simulink model "add_entry_model"  (R2020b)
settings: Solver=FixedStepDiscrete  StartTime=0.0  StopTime=0.1  FixedStep=0.1  RelTol=1e-3
undefined symbols (not defined in the file or in its folder): kConsecutiveIndexDelta, kContainerLength, test_input
libraries: move_index_lib x2
settings Model: Creator=rsub  LastModifiedBy=rsub

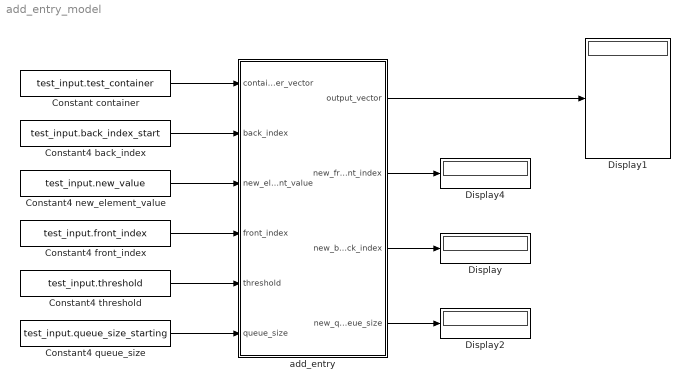
== system add_entry_model ==
  Constant container : Constant  Value=test_input.test_container
  Constant4 back_index : Constant  Value=test_input.back_index_start
  Constant4 front_index : Constant  Value=test_input.front_index
  Constant4 new_element_value : Constant  Value=test_input.new_value
  Constant4 queue_size : Constant  Value=test_input.queue_size_starting
  Constant4 threshold : Constant  Value=test_input.threshold
  Display{,1..2,4} (4 alike) : Display
  add_entry : Subsystem
  wires:
  Constant container/1 -> add_entry/1(container_vector)
  Constant4 back_index/1 -> add_entry/2(back_index)
  Constant4 new_element_value/1 -> add_entry/3(new_element_value)
  add_entry/1(output_vector) -> Display1/1
  add_entry/3(new_back_index) -> Display/1
  Constant4 front_index/1 -> add_entry/4(front_index)
  Constant4 threshold/1 -> add_entry/5(threshold)
  Constant4 queue_size/1 -> add_entry/6(queue_size)
  add_entry/2(new_front_index) -> Display4/1
  add_entry/4(new_queue_size) -> Display2/1

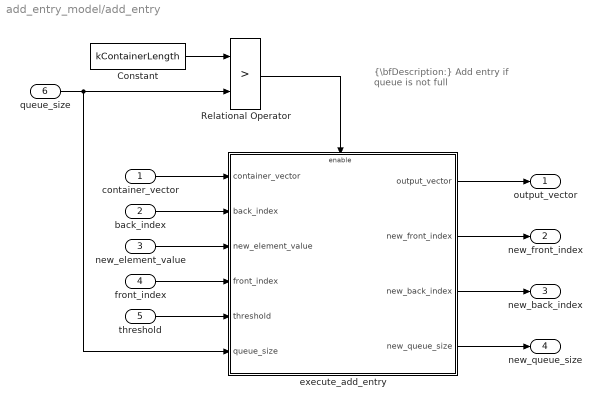
== system add_entry_model/add_entry ==
  note: {\bfDescription:}
      | Add entry if queue is not full
  container_vector : Inport
  back_index : Inport  Port=2
  new_element_value : Inport  Port=3
  front_index : Inport  Port=4
  threshold : Inport  Port=5
  queue_size : Inport  Port=6
  Constant : Constant  Value=kContainerLength
  Relational Operator : RelationalOperator  Operator=>  OutDataTypeStr=boolean  RndMeth=Simplest
  execute_add_entry : Subsystem
  output_vector : Outport
  new_front_index : Outport  Port=2
  new_back_index : Outport  Port=3
  new_queue_size : Outport  Port=4
  wires:
  container_vector/1 -> execute_add_entry/1(container_vector)
  back_index/1 -> execute_add_entry/2(back_index)
  new_element_value/1 -> execute_add_entry/3(new_element_value)
  front_index/1 -> execute_add_entry/4(front_index)
  threshold/1 -> execute_add_entry/5(threshold)
  queue_size/1 -> execute_add_entry/6(queue_size), Relational Operator/2
  execute_add_entry/1(output_vector) -> output_vector/1
  execute_add_entry/2(new_front_index) -> new_front_index/1
  execute_add_entry/3(new_back_index) -> new_back_index/1
  execute_add_entry/4(new_queue_size) -> new_queue_size/1
  Constant/1 -> Relational Operator/1
  Relational Operator/1 -> execute_add_entry/Enable

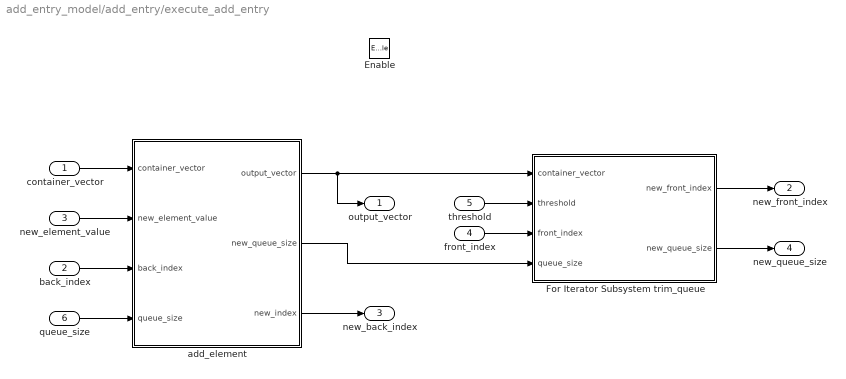
== system add_entry_model/add_entry/execute_add_entry ==
  container_vector : Inport
  back_index : Inport  Port=2
  new_element_value : Inport  Port=3
  front_index : Inport  Port=4
  threshold : Inport  Port=5
  queue_size : Inport  Port=6
  Enable : EnablePort
  For Iterator Subsystem trim_queue : Subsystem  TreatAsAtomicUnit=on
  add_element : Subsystem
  output_vector : Outport  InitialOutput=test_input.test_container
  new_front_index : Outport  Port=2  InitialOutput=test_input.front_index
  new_back_index : Outport  Port=3  InitialOutput=test_input.back_index_start
  new_queue_size : Outport  Port=4  InitialOutput=test_input.queue_size_starting
  wires:
  threshold/1 -> For Iterator Subsystem trim_queue/2(threshold)
  new_element_value/1 -> add_element/2(new_element_value)
  For Iterator Subsystem trim_queue/1(new_front_index) -> new_front_index/1
  container_vector/1 -> add_element/1(container_vector)
  add_element/3(new_index) -> new_back_index/1
  back_index/1 -> add_element/3(back_index)
  front_index/1 -> For Iterator Subsystem trim_queue/3(front_index)
  add_element/2(new_queue_size) -> For Iterator Subsystem trim_queue/4(queue_size)
  For Iterator Subsystem trim_queue/2(new_queue_size) -> new_queue_size/1
  queue_size/1 -> add_element/4(queue_size)
  add_element/1(output_vector) -> output_vector/1, For Iterator Subsystem trim_queue/1(container_vector)

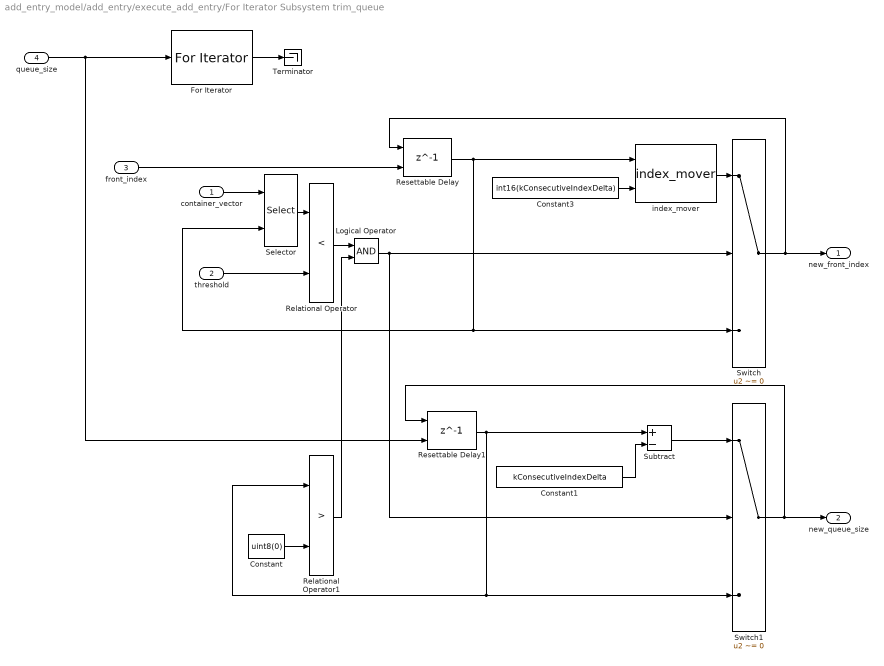
== system add_entry_model/add_entry/execute_add_entry/For Iterator Subsystem trim_queue ==
  container_vector : Inport
  threshold : Inport  Port=2
  front_index : Inport  Port=3
  queue_size : Inport  Port=4
  Constant : Constant  Value=uint8(0)
  Constant1 : Constant  Value=kConsecutiveIndexDelta
  Constant3 : Constant  Value=int16(kConsecutiveIndexDelta)
  For Iterator : ForIterator  IterationSource=external  IterationLimit=kContainerLength  IndexMode=Zero-based  IterationVariableDataType=uint8
  Logical Operator : Logic  AllPortsSameDT=off  OutDataTypeStr=boolean
  Relational Operator : RelationalOperator  Operator=<  OutDataTypeStr=boolean  RndMeth=Simplest
  Relational Operator1 : RelationalOperator  Operator=>  OutDataTypeStr=boolean  RndMeth=Simplest
  Resettable Delay : Delay  DelayLength=1  InitialConditionSource=Input port
      settings: InputPortMap=u0,p4
  Resettable Delay1 : Delay  DelayLength=1  InitialConditionSource=Input port
      settings: InputPortMap=u0,p4
  Selector : Selector  IndexMode=Zero-based  InputPortWidth=kContainerLength  IndexOptions=Index vector (port)  Indices=[1 3]  OutputSizes=1
  Subtract : Sum  Inputs=+-
  Switch : Switch  Criteria=u2 ~= 0
  Switch1 : Switch  Criteria=u2 ~= 0
  Terminator : Terminator
  index_mover : move_index_lib/index_mover  SystemSampleTime=-1  VariantActivationTime=update diagram  Latency=0  AutoFrameSizeCalculation=off
  new_front_index : Outport
  new_queue_size : Outport  Port=2
  wires:
  queue_size/1 -> Resettable Delay1/2, For Iterator/1
  For Iterator/1 -> Terminator/1
  container_vector/1 -> Selector/1
  front_index/1 -> Resettable Delay/2
  Selector/1 -> Relational Operator/1
  threshold/1 -> Relational Operator/2
  Logical Operator/1 -> Switch/2, Switch1/2
  Switch/1 -> Resettable Delay/1, new_front_index/1
  index_mover/1 -> Switch/1
  Constant3/1 -> index_mover/2
  Resettable Delay/1 -> Switch/3, Selector/2, index_mover/1
  Switch1/1 -> new_queue_size/1, Resettable Delay1/1
  Resettable Delay1/1 -> Switch1/3, Relational Operator1/1, Subtract/1
  Subtract/1 -> Switch1/1
  Constant1/1 -> Subtract/2
  Relational Operator/1 -> Logical Operator/1
  Constant/1 -> Relational Operator1/2
  Relational Operator1/1 -> Logical Operator/2

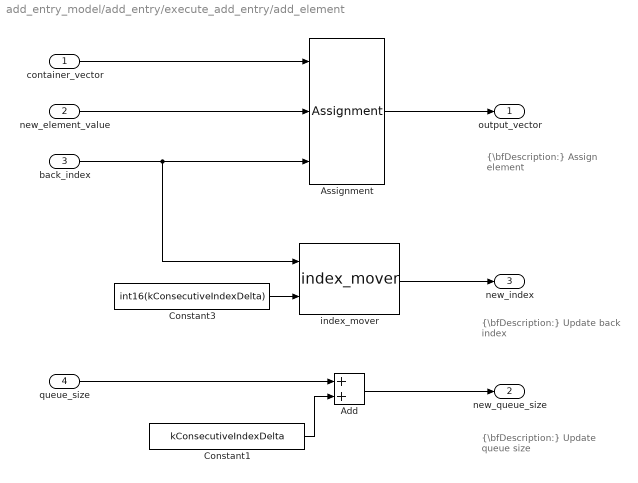
== system add_entry_model/add_entry/execute_add_entry/add_element ==
  note: {\bfDescription:}
      | Assign element
  note: {\bfDescription:}
      | Update back index
  note: {\bfDescription:}
      | Update queue size
  container_vector : Inport
  new_element_value : Inport  Port=2
  back_index : Inport  Port=3
  queue_size : Inport  Port=4
  Add : Sum
  Assignment : Assignment  IndexMode=Zero-based  DiagnosticForDimensions=Warning  IndexOptions=Index vector (port)  Indices=1  OutputSizes=1
  Constant1 : Constant  Value=kConsecutiveIndexDelta
  Constant3 : Constant  Value=int16(kConsecutiveIndexDelta)
  index_mover : move_index_lib/index_mover  SystemSampleTime=-1  VariantActivationTime=update diagram  Latency=0  AutoFrameSizeCalculation=off
  output_vector : Outport
  new_queue_size : Outport  Port=2
  new_index : Outport  Port=3
  wires:
  new_element_value/1 -> Assignment/2
  container_vector/1 -> Assignment/1
  Constant3/1 -> index_mover/2
  queue_size/1 -> Add/1
  Constant1/1 -> Add/2
  Assignment/1 -> output_vector/1
  back_index/1 -> index_mover/1, Assignment/3
  index_mover/1 -> new_index/1
  Add/1 -> new_queue_size/1
